simulink model "EL_Circuit"  (R2012b)
settings: Solver=ode15s  StartTime=0.0  StopTime=.1  FixedStep=1e-4  RelTol=1e-6
settings Model: Creator=David  LastModifiedBy=David
settings DataIOCC: SignalLoggingSaveFormat=ModelDataLogs
settings DebuggingCC: FcnCallInpInsideContextMsg=UseLocalSettings
settings RTWCC: TargetLang=C++
settings GRTTargetCC: CombineOutputUpdateFcns=off  GRTInterface=on

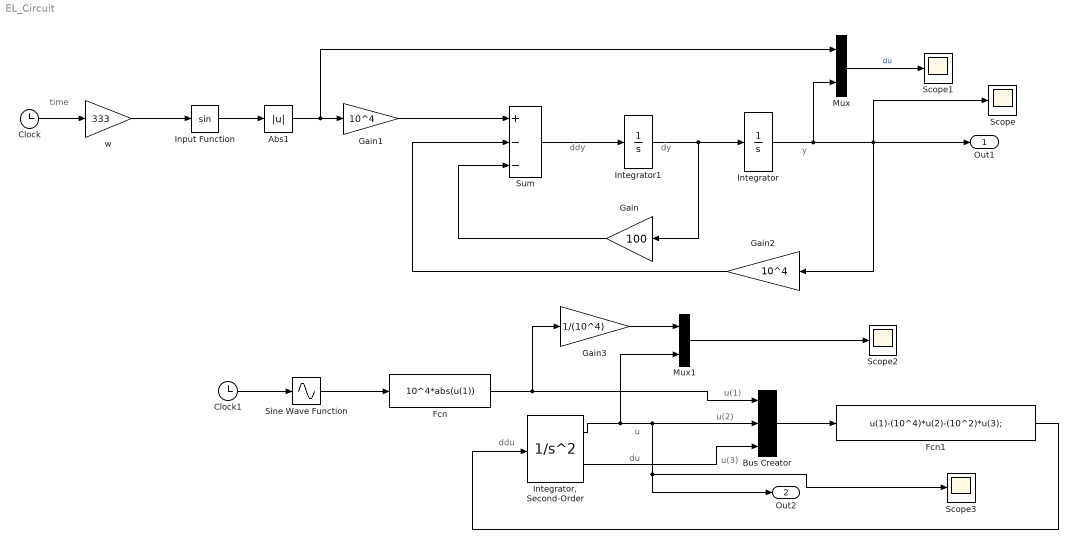
== system EL_Circuit ==
  note: ddy
  note: dy
  note: y
  note: u
  note: du
  note: ddu
  note: u(1)
  note: u(2)
  note: u(3)
  note: time
  Abs1 : Abs
  Bus Creator : BusCreator  Inputs=3
  Clock : Clock
  Clock1 : Clock
  Fcn : Fcn  Expr=10^4*abs(u(1))
  Fcn1 : Fcn  Expr=u(1)-(10^4)*u(2)-(10^2)*u(3);
  Gain : Gain  Gain=100
  Gain1 : Gain  Gain=10^4
  Gain2 : Gain  Gain=10^4
  Gain3 : Gain  Gain=1/(10^4)
  Input Function : Trigonometry
  Integrator : Integrator
  "Integrator, Second-Order" : SecondOrderIntegrator
  Integrator1 : Integrator
  Mux : Mux  Inputs=2
  Mux1 : Mux  Inputs=2
  Scope{,1..3} (4 alike) : Scope
      Scope2 settings: SaveName=ScopeData2
      Scope3 settings: SaveName=ScopeData3
  Sine Wave Function : Sin  TimeSource=Use external signal  Frequency=333  SampleTime=0
  Sum : Sum  Inputs=+--
  w : Gain  Gain=333
  Out1 : Outport
  Out2 : Outport  Port=2
  wires:
  Input Function/1 -> Abs1/1
  Abs1/1 -> Gain1/1, Mux/1
  Gain1/1 -> Sum/1
  Sum/1 -> Integrator1/1
  Integrator1/1 -> Integrator/1, Gain/1
  Integrator/1 -> Out1/1, Scope/1, Gain2/1, Mux/2
  Gain/1 -> Sum/3
  Gain2/1 -> Sum/2
  Mux/1 -> Scope1/1  "du"
  w/1 -> Input Function/1
  Clock/1 -> w/1
  Clock1/1 -> Sine Wave Function/1
  Sine Wave Function/1 -> Fcn/1
  Fcn/1 -> Gain3/1, Bus Creator/1
  Fcn1/1 -> "Integrator, Second-Order"/1
  "Integrator, Second-Order"/1 -> Mux1/2, Bus Creator/2, Out2/1, Scope3/1
  "Integrator, Second-Order"/2 -> Bus Creator/3
  Mux1/1 -> Scope2/1
  Bus Creator/1 -> Fcn1/1
  Gain3/1 -> Mux1/1
